simulink model "impedanceControl"  (R2018b)
settings: Solver=VariableStepAuto  StartTime=0.0  StopTime=7  RelTol=1e-3
values from neighbouring files (symbols this model uses):
  Bd = 1    [matlab.mat]
  Kb = 0.00416666666667    [matlab.mat]
  Kd = 3    [matlab.mat]
  Kt = 0.0398    [matlab.mat]
  L = 0.000281    [matlab.mat]
  Md = 1    [matlab.mat]
  R = 1.45    [matlab.mat]
  Te = 0.0096837944664    [matlab.mat]
  Th = 1    [matlab.mat]
libraries: simulink x1
settings Model: Creator=DELL  LastModifiedBy=holyCow

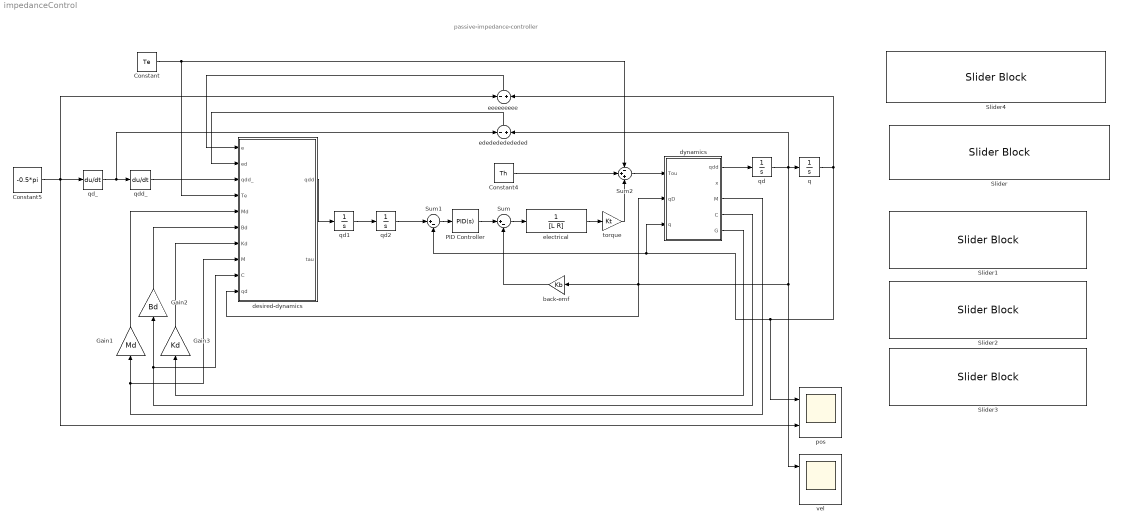
== system impedanceControl ==
  note: passive-impedance-controller
  Constant : Constant  Value=Te
  Constant4 : Constant  Value=Th
  Constant5 : Constant  Value=-0.5*pi
  Gain1 : Gain  Gain=Md
  Gain2 : Gain  Gain=Bd
  Gain3 : Gain  Gain=Kd
  PID Controller : simulink/Continuous/PID Controller  Controller=PID  Form=Parallel  TimeDomain=Continuous-time  SampleTime=-1  IntegratorMethod=Forward Euler  FilterMethod=Forward Euler  ControllerParametersSource=internal  P=7.88491030804892e-06  I=4.91012552196856e-08  D=0.000301677021149975  UseFilter=on  N=0.397462247961043  TunerSelectOption=Transfer Function Based (PID Tuner App)  InitialConditionSource=internal  InitialConditionForIntegrator=0  InitialConditionForFilter=0  DifferentiatorICPrevScaledInput=0  ExternalReset=none  TrackingMode=off  Kt=1  LimitOutput=off  UpperSaturationLimit=inf  LowerSaturationLimit=-inf  LinearizeAsGain=on  AntiWindupMode=none  Kb=1  POutMin=[]  POutMax=[]  IOutMin=[]  IOutMax=[]  DOutMin=[]  DOutMax=[]  NOutMin=[]  NOutMax=[]  SumOutMin=[]  SumOutMax=[]  SaturationOutMin=[]  SaturationOutMax=[]  PParamMin=[]  PParamMax=[]  IParamMin=[]  IParamMax=[]  DParamMin=[]  DParamMax=[]  NParamMin=[]  NParamMax=[]  KbParamMin=[]  KbParamMax=[]  KtParamMin=[]  KtParamMax=[]  KbOutMin=[]  KbOutMax=[]  KtOutMin=[]  KtOutMax=[]  IntegratorOutMin=[]  IntegratorOutMax=[]  FilterOutMin=[]  FilterOutMax=[]  SumI1OutMin=[]  SumI1OutMax=[]  SumI2OutMin=[]  SumI2OutMax=[]  SumI3OutMin=[]  SumI3OutMax=[]  SumI4OutMin=[]  SumI4OutMax=[]  SumDOutMin=[]  SumDOutMax=[]  DifferentiatorOutMin=[]  DifferentiatorOutMax=[]  FilterDiffOutCoefMin=[]  FilterDiffOutCoefMax=[]  ReciprocalOutMin=[]  ReciprocalOutMax=[]  SumDenOutMin=[]  SumDenOutMax=[]  SumNumOutMin=[]  SumNumOutMax=[]  DivideOutMin=[]  DivideOutMax=[]  IntegratorContinuousStateAttributes=''  IntegratorStateMustResolveToSignalObject=off  IntegratorRTWStateStorageClass=Auto  FilterContinuousStateAttributes=''  FilterStateMustResolveToSignalObject=off  FilterRTWStateStorageClass=Auto  ParallelPVariant=InternalParameters  IdealPVariant=Disabled  IVariant=InternalParameters  DVariant=InternalParameters  IntegratorVariant=Continuous  SatVariant=Disabled  AWVariant=Passthrough  PCopyVariant=Disabled  TRVariant=Disabled  FdbkBlocksVariant=Forward  IdealPFdbkVariant=Disabled  SatFdbkVariant=Disabled  DerivativeFilterVariant=ContFilter  NVariant=InternalParameters  NCopyVariant=Disabled  FilterICVariant=InternalICsFilter  IntegratorICVariant=InternalICs  ExternalResetVariant=Disabled  TRSumVariant=Passthrough  SumFdbkVariant=Disabled  SumVariant=Sum_PID
  Slider : SliderBlock  WebBlockId=98  ScaleMax=2
  Slider1 : SliderBlock  WebBlockId=99  ScaleMax=2
  Slider2 : SliderBlock  WebBlockId=103  ScaleMax=2
  Slider3 : SliderBlock  WebBlockId=104  ScaleMax=2
  Slider4 : SliderBlock  WebBlockId=111  ScaleMax=1
  Sum : Sum  Inputs=|+-
  Sum1 : Sum  Inputs=|+-
  Sum2 : Sum  Inputs=-++
  "back-emf " : Gain  Gain=Kb
  desired-dynamics : MATLAB Function  TreatAsAtomicUnit=on
  dynamics : MATLAB Function  TreatAsAtomicUnit=on
  ededededededed : Sum  Inputs=-+
  eeeeeeeee : Sum  Inputs=-+
  electrical : TransferFcn  Denominator=[L R]
  pos : Scope  NumInputPorts=2
  q : Integrator
  qd : Integrator
  qd1 : Integrator
  qd2 : Integrator
  "qd_ " : Derivative
  qdd_ : Derivative
  torque : Gain  Gain=Kt
  vel : Scope  NumInputPorts=2
  wires:
  electrical/1 -> torque/1
  torque/1 -> Sum2/3
  "back-emf "/1 -> Sum/2
  PID Controller/1 -> Sum/1
  Sum/1 -> electrical/1
  Sum1/1 -> PID Controller/1
  desired-dynamics/1(qdd) -> qd1/1
  dynamics/3(M) -> Gain1/1, desired-dynamics/8(M)
  dynamics/4(C) -> desired-dynamics/9(C), Gain2/1
  Gain1/1 -> desired-dynamics/5(Md)
  Gain2/1 -> desired-dynamics/6(Bd)
  dynamics/5(G) -> Gain3/1
  Gain3/1 -> desired-dynamics/7(Kd)
  Constant5/1 -> eeeeeeeee/1, "qd_ "/1, pos/2
  qd/1 -> "back-emf "/1, dynamics/2(qD), desired-dynamics/10(qd), vel/1, ededededededed/2, q/1
  qdd_/1 -> desired-dynamics/3(qdd_)
  q/1 -> Sum1/2, dynamics/3(q), pos/1, eeeeeeeee/2
  eeeeeeeee/1 -> desired-dynamics/1(e)
  ededededededed/1 -> desired-dynamics/2(ed)
  Constant/1 -> desired-dynamics/4(Te), Sum2/1
  Sum2/1 -> dynamics/1(Tou)
  Constant4/1 -> Sum2/2
  dynamics/1(qdd) -> qd/1
  qd1/1 -> qd2/1
  qd2/1 -> Sum1/1
  "qd_ "/1 -> ededededededed/1, qdd_/1

== matlab function impedanceControl/desired-dynamics ==
  data: e input; ed input; qdd_ input; Te input; Md input; Bd input; Kd input; M input; C input; qd input; qdd output; tau output
function [qdd, tau]= fcn(e, ed, qdd_, Te, Md, Bd, Kd, M, C, qd)
qdd = qdd_ - (Bd*ed + Kd - Te)/Md;
tau = C*ed + G + M*qdd;

== matlab function impedanceControl/dynamics ==
  data: Tou input; qD input; qdd output; q input; x output; M output; C output; G output
function [qdd, x, M, C, G]= fcn(Tou, qD, q)
l = 0.265;
m = 0.170;
a = 0.110;
b = 0.090;

g = 9.81;

m1 = 2.5;
m2 = 0.2;
%mr = 0.1;
mf = 0.075;

% measure of radius
rr = 0.110/2;
rf = 0.075/2;

delta = rr - rf;

% l*sin(q2) + delta = m*sin(q1 - q2)
ta = (l/m + cos(q))^2 + (sin(q))^2;
tb = -2*(delta/m)*sin(q);
tc = (delta/m)^2 - (l/m + cos(q))^2;

q2 = acos((-tb + sqrt(tb^2 - 4*ta*tc))/(2*ta));
k = 1/(1 + ((l*cos(q2))/(m*cos(q - q2))));
%q2D = k * q1D;

x = sqrt(l^2 + m^2 - delta^2 + 2*l*m*cos(q));
c = ((-l*m*sin(q))/x);
%xD = c * q1D;

s = (l*k*m*sin(q2)*cos(q - q2) - l*m*cos(q2)*sin(q - q2)*(1 - k))/((l*cos(q2) + m*cos(q - q2))^2);
u = (l*m*(c*sin(q) - x*cos(q)))/(x^2);

%kD = s * q1D;
%cD = u * q1D;

%xa = a*cos(q2);
%xaD = -a*sin(q2)*q2D;

%ya = rr + a*sin(q2);
%yaD = a*cos(q2)*q2D;

%xb = x - b*cos(q1 - q2);
%xbD = xD + b*sin(q1 - q2)*(q1D - q2D);

%yb = rf + b*sin(q1 - q2);
%ybD = b*cos(q1 - q2)*(q1D - q2D);

%K = 0.5*m1*(xaD^2 + yaD^2) + 0.5*m2*(xbD^2 + ybD^2) + 0.75*mf*xD^2;
%P = mr*g*rr + mf*g*rf + m1*g*ya + m2*g*yb;

M = m1*(a^2)*(k^2) + (m2 + 1.5*mf)*(c^2) + m2*(b^2)*((1-k)^2) + 2*m2*b*sin(q - q2)*c*(1-k);

ctemp = cos(q - q2)*c*((1-k)^2) + sin(q - q2)*u*(1-k) - sin(q - q2)*c*s;
C = (m1*(a^2)*k*s + (m2 + 1.5*mf)*c*u - m2*(b^2)*s*(1-k) + m2*b*ctemp) * (qD);

G = m1*g*a*cos(q2)*k + m2*g*b*cos(q - q2)*(1 - k);
qdd = (Tou - C*qD - G)/M;
